simulink library "Euler_to_DCM_lib"  (Simulink 6.6)
libraries: simulink x1
settings Model: Creator=cbuttril  LastModifiedBy=cbuttril

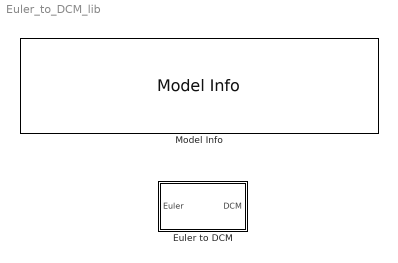
== system Euler_to_DCM_lib ==
  Euler to DCM : Subsystem
  Model Info : simulink/Model-Wide Utilities/Model Info  SystemSampleTime=-1  InitialBlockCM=None  BlockCM=None  Frame=on  DisplayStringWithTags=|  HorizontalTextAlignment=Center  LeftAlignmentValue=0.5  SourceBlockDiagram=Euler_to_DCM_lib  TagMaxNumber=20
      | Developed using Matlab Release 2007a
      | 
      | SVN:%<ModelVersion>
      | Last modifed by %<LastModifiedBy> on %<LastModificationDate>

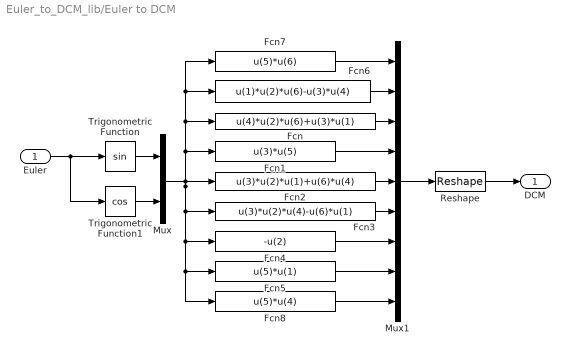
== system Euler_to_DCM_lib/Euler to DCM ==
  "Euler " : Inport
  Fcn : Fcn  Expr=u(4)*u(2)*u(6)+u(3)*u(1)
  Fcn1 : Fcn  Expr=u(3)*u(5)
  Fcn2 : Fcn  Expr=u(3)*u(2)*u(1)+u(6)*u(4)
  Fcn3 : Fcn  Expr=u(3)*u(2)*u(4)-u(6)*u(1)
  Fcn4 : Fcn  Expr=-u(2)
  Fcn5 : Fcn  Expr=u(5)*u(1)
  Fcn6 : Fcn  Expr=u(1)*u(2)*u(6)-u(3)*u(4)
  Fcn7 : Fcn  Expr=u(5)*u(6)
  Fcn8 : Fcn  Expr=u(5)*u(4)
  Mux : Mux  Inputs=2
  Mux1 : Mux  Inputs=9
  Reshape : Reshape  OutputDimensionality=Customize  OutputDimensions=[3,3]
  Trigonometric Function : Trigonometry
  Trigonometric Function1 : Trigonometry  Operator=cos
  DCM : Outport
  wires:
  Reshape/1 -> DCM/1
  Fcn8/1 -> Mux1/9
  Fcn5/1 -> Mux1/8
  Fcn4/1 -> Mux1/7
  Fcn3/1 -> Mux1/6
  Fcn2/1 -> Mux1/5
  Fcn1/1 -> Mux1/4
  Fcn/1 -> Mux1/3
  Fcn6/1 -> Mux1/2
  Fcn7/1 -> Mux1/1
  Mux1/1 -> Reshape/1
  Mux/1 -> Fcn3/1, Fcn5/1, Fcn8/1, Fcn4/1, Fcn2/1, Fcn1/1, Fcn6/1, Fcn7/1, Fcn/1
  Trigonometric Function1/1 -> Mux/2
  Trigonometric Function/1 -> Mux/1
  "Euler "/1 -> Trigonometric Function/1, Trigonometric Function1/1
